simulink model "pedal_project"  (R2025b)
settings: Solver=VariableStepAuto  StartTime=0.0  StopTime=10.0  RelTol=1e-3
(part 2 of 2)

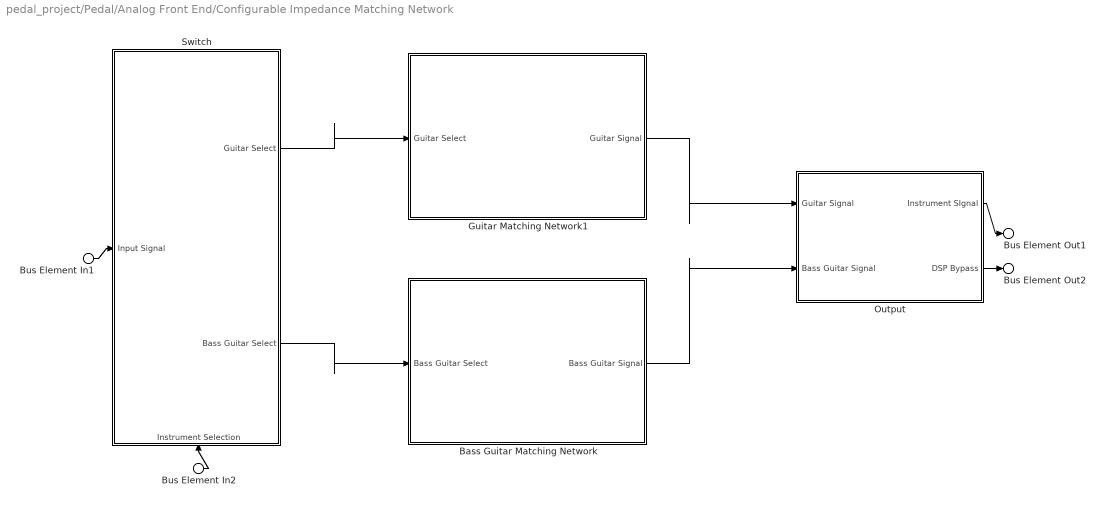
== system pedal_project/Pedal/Analog Front End/Configurable Impedance Matching Network ==
  Bus Element In2 : Inport  PortName=Instrument Selection
  Bus Element In1 : Inport  Port=2  PortName=Input Signal
  Bass Guitar Matching Network : Subsystem
      settings: PortSchema="{\"entries\":[{\"content\":{\"headerSize\":26,\"margin\":15,\"minimumSpacing\":25,\"sides\":[{\"content\":{\"connectorIds\":[\"In1\"]},\"type\":\"ConnectorPlacement.EquallySpacedRectSide\",\"uuid\":\"d45e420a-c48a-4f64-96ce-c5c35bb4ca1a\"},{\"content\":{\"connectorIds\":[\"Out1\"],\"side\":\"RIGHT\"},\"type\":\"ConnectorPlacement.EquallySpacedRectSide\",\"uuid\":\"a4e2bce0-d957-4e8d-907b-26e945724fec\"},{\"content\":{\"side\":\"TOP\"},\"type\":\"ConnectorPlacement.EquallySpacedRectSide\",\"uuid\":\"f887741f-84ea-4dc9-b916-61633ba77119\"}]},\"type\":\"ConnectorPlacement.EquallySpacedConnector\",\"uuid\":\"ffda6ec7-3a8c-4734-85c7-d4d2baf408ab\"}],\"packageUris\":[\"http://schema.mathworks.com/mf0/Connector/R2020b\"],\"version\":\"1.0\"}"
  Guitar Matching Network1 : Subsystem
      settings: PortSchema="{\"entries\":[{\"content\":{\"headerSize\":26,\"margin\":15,\"minimumSpacing\":25,\"sides\":[{\"content\":{\"connectorIds\":[\"In1\"]},\"type\":\"ConnectorPlacement.EquallySpacedRectSide\",\"uuid\":\"d45e420a-c48a-4f64-96ce-c5c35bb4ca1a\"},{\"content\":{\"connectorIds\":[\"Out1\"],\"side\":\"RIGHT\"},\"type\":\"ConnectorPlacement.EquallySpacedRectSide\",\"uuid\":\"a4e2bce0-d957-4e8d-907b-26e945724fec\"},{\"content\":{\"side\":\"TOP\"},\"type\":\"ConnectorPlacement.EquallySpacedRectSide\",\"uuid\":\"f887741f-84ea-4dc9-b916-61633ba77119\"}]},\"type\":\"ConnectorPlacement.EquallySpacedConnector\",\"uuid\":\"ffda6ec7-3a8c-4734-85c7-d4d2baf408ab\"}],\"packageUris\":[\"http://schema.mathworks.com/mf0/Connector/R2020b\"],\"version\":\"1.0\"}"
  Output : Subsystem
      settings: PortSchema="{\"entries\":[{\"content\":{\"headerSize\":26,\"margin\":15,\"minimumSpacing\":25,\"sides\":[{\"content\":{\"connectorIds\":[\"In1\",\"In2\"]},\"type\":\"ConnectorPlacement.EquallySpacedRectSide\",\"uuid\":\"d45e420a-c48a-4f64-96ce-c5c35bb4ca1a\"},{\"content\":{\"connectorIds\":[\"Out1\",\"Out2\"],\"side\":\"RIGHT\"},\"type\":\"ConnectorPlacement.EquallySpacedRectSide\",\"uuid\":\"a4e2bce0-d957-4e8d-907b-26e945724fec\"},{\"content\":{\"side\":\"TOP\"},\"type\":\"ConnectorPlacement.EquallySpacedRectSide\",\"uuid\":\"f887741f-84ea-4dc9-b916-61633ba77119\"}]},\"type\":\"ConnectorPlacement.EquallySpacedConnector\",\"uuid\":\"ffda6ec7-3a8c-4734-85c7-d4d2baf408ab\"}],\"packageUris\":[\"http://schema.mathworks.com/mf0/Connector/R2020b\"],\"version\":\"1.0\"}"
  Switch : Subsystem
      settings: PortSchema="{\"entries\":[{\"content\":{\"headerSize\":26,\"margin\":15,\"minimumSpacing\":25,\"sides\":[{\"content\":{\"connectorIds\":[\"In2\"]},\"type\":\"ConnectorPlacement.EquallySpacedRectSide\",\"uuid\":\"d45e420a-c48a-4f64-96ce-c5c35bb4ca1a\"},{\"content\":{\"connectorIds\":[\"Out1\",\"Out2\"],\"side\":\"RIGHT\"},\"type\":\"ConnectorPlacement.EquallySpacedRectSide\",\"uuid\":\"a4e2bce0-d957-4e8d-907b-26e945724fec\"},{\"content\":{\"side\":\"TOP\"},\"type\":\"ConnectorPlacement.EquallySpacedRectSide\",\"uuid\":\"f887741f-84ea-4dc9-b916-61633ba77119\"},{\"content\":{\"connectorIds\":[\"In1\"],\"side\":\"BOTTOM\"},\"type\":\"ConnectorPlacement.EquallySpacedRectSide\",\"uuid\":\"dfd7a217-587e-4736-a22e-6266921a1acc\"}]},\"type\":\"ConnectorPlacement.EquallySpacedConnector\",\"uuid\":\"ffda6ec7-3a8c-4734-85c7-d4d2baf408ab\"}],\"packageUris\":[\"http://schema.mathworks.com/mf0/Connector/R2020b\"],\"version\":\"1.0\"}"
  Bus Element Out1 : Outport  PortName=Instrument SIgnal
  Bus Element Out2 : Outport  Port=2  PortName=DSP Bypass
  wires:
  Bus Element In1/1 -> Switch/2(Input Signal)
  Switch/1(Guitar Select) -> Guitar Matching Network1/1(Guitar Select)
  Switch/2(Bass Guitar Select) -> Bass Guitar Matching Network/1(Bass Guitar Select)
  Bus Element In2/1 -> Switch/1(Instrument Selection)
  Output/1(Instrument SIgnal) -> Bus Element Out1/1
  Guitar Matching Network1/1(Guitar Signal) -> Output/1(Guitar Signal)
  Bass Guitar Matching Network/1(Bass Guitar Signal) -> Output/2(Bass Guitar Signal)
  Output/2(DSP Bypass) -> Bus Element Out2/1

== system pedal_project/Pedal/Analog Signal Processing/1//4 Inch TS Input Jack1 ==
  Bus Element In1 : Inport  PortName=Post Extern Sig
  Bus Element Out1 : Outport  PortName=External Signal

== system pedal_project/Pedal/Analog Signal Processing/1//4 Inch TS Ouput Jack ==
  Bus Element In1 : Inport  PortName=Extern Sig Input
  Bus Element Out1 : Outport  PortName=Post DSP Sig

== system pedal_project/Pedal/Analog Signal Processing/Analog Processing Network ==
  Bus Element In3 : Inport  PortName=Post Extern Sig
  Bus Element In1 : Inport  Port=2  PortName=ASP Effects Power
  Bus Element In2 : Inport  Port=3  PortName=Analog Chain Config
  Bus Element Out1 : Outport  PortName=Post ASP Sig

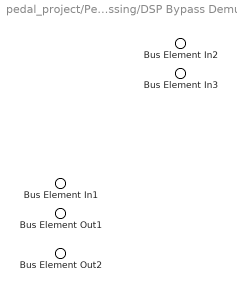
== system pedal_project/Pedal/Analog Signal Processing/DSP Bypass Demux ==
  Bus Element In3 : Inport  PortName=DSP Bypass Config
  Bus Element In2 : Inport  Port=2  PortName=DSP Bypass
  Bus Element In1 : Inport  Port=3  PortName=DSP Signal
  Bus Element Out1 : Outport  PortName=Extern Sig Input
  Bus Element Out2 : Outport  Port=2  PortName=Extern Bypass Sig

== system pedal_project/Pedal/Analog Signal Processing/Extern Bypass Demux ==
  Bus Element In2 : Inport  PortName=Extern Bypass Sig
  Bus Element In1 : Inport  Port=2  PortName=External Signal
  Bus Element Out1 : Outport  PortName=Post Extern Sig

== system pedal_project/Pedal/Control/Dial//Switch Network ==
  Bus Element Out1 : Outport  PortName=Parameters Config

== system pedal_project/Pedal/Control/Input Type Selector ==
  Bus Element Out1 : Outport  PortName=Instrument Selection

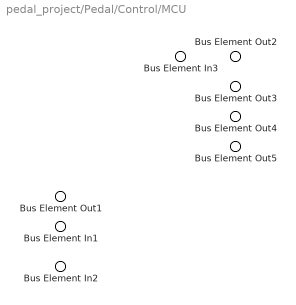
== system pedal_project/Pedal/Control/MCU ==
  Bus Element In3 : Inport  PortName=MCU Power
  Bus Element In1 : Inport  Port=2  PortName=Parameters Config
  Bus Element In2 : Inport  Port=3  PortName=Configuration Packets
  Bus Element Out5 : Outport  PortName=ASP Bypass Config
  Bus Element Out4 : Outport  Port=2  PortName=Preamp Bypass
  Bus Element Out3 : Outport  Port=3  PortName=DSP Bypass Config
  Bus Element Out2 : Outport  Port=4  PortName=Analog Chain Config
  Bus Element Out1 : Outport  Port=5  PortName=DSP Config

== system pedal_project/Pedal/Control/USB Port ==
  Bus Element In1 : Inport  PortName=App Control Packets
  Bus Element Out1 : Outport  PortName=Configuration Packets

== system pedal_project/Pedal/Digital Signal Processing/40 kHz LPF ==
  Bus Element In1 : Inport  PortName=DSP Output Sig
  Bus Element Out1 : Outport  PortName=DSP Signal
  Bus Element Out2 : Outport  Port=2  PortName=ASP Bypass

== system pedal_project/Pedal/Digital Signal Processing/DSP Core ==
  Bus Element In3 : Inport  PortName=DSP Config
  Bus Element In2 : Inport  Port=2  PortName=DSP Core Power
  Bus Element In1 : Inport  Port=3  PortName=Instrument SIgnal
  Bus Element Out1 : Outport  PortName=DSP Output Sig

== system pedal_project/Pedal/Electronics Power Distribution/9V 2.1mm Jack ==
  Bus Element In1 : Inport  PortName=9V DC
  Bus Element Out1 : Outport  PortName=DC In

== system pedal_project/Pedal/Electronics Power Distribution/Power Bus ==
  Bus Element In1 : Inport  PortName=DC In
  Bus Element Out2 : Outport  PortName=DSP Core Power
  Bus Element Out3 : Outport  Port=2  PortName=ASP Effects Power
  Bus Element Out1 : Outport  Port=3  PortName=MCU Power

== system pedal_project/Pedal/Output Drivers/1//4 Inch TS Ouput ==
  Bus Element In1 : Inport  PortName=Amp Sig
  Bus Element Out1 : Outport  PortName=TS Out

== system pedal_project/Pedal/Output Drivers/1//8 Inch TRS Ouput ==
  Bus Element In1 : Inport  PortName=Amp TRS Sig
  Bus Element Out1 : Outport  PortName=TRS Out

== system pedal_project/Pedal/Output Drivers/ASP Bypass Demux ==
  Bus Element In3 : Inport  PortName=ASP Bypass Config
  Bus Element In2 : Inport  Port=2  PortName=Post ASP Sig
  Bus Element In1 : Inport  Port=3  PortName=ASP Bypass
  Bus Element Out1 : Outport  PortName=ASP Sig

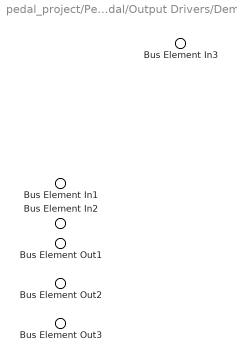
== system pedal_project/Pedal/Output Drivers/Demux ==
  Bus Element In1 : Inport  PortName=Amplified Signal
  Bus Element In3 : Inport  Port=2  PortName=Bypass Sig
  Bus Element In2 : Inport  Port=3  PortName=Preamp Bypass
  Bus Element Out1 : Outport  PortName=Amp TS Sig
  Bus Element Out2 : Outport  Port=2  PortName=Amp XLR Sig
  Bus Element Out3 : Outport  Port=3  PortName=Amp TRS Sig

== system pedal_project/Pedal/Output Drivers/Out Bus ==
  Bus Element In4 : Inport  PortName=MIDI Sig
  Bus Element In1 : Inport  Port=2  PortName=TS Out
  Bus Element In2 : Inport  Port=3  PortName=XLR Out
  Bus Element In3 : Inport  Port=4  PortName=TRS Out
  Bus Element Out1 : Outport  PortName=Audio Signal Output

== system pedal_project/Pedal/Output Drivers/Preamp ==
  Bus Element In1 : Inport  PortName=Preamp Sig
  Bus Element Out1 : Outport  PortName=Amplified Signal

== system pedal_project/Pedal/Output Drivers/Sig Combiner ==
  Bus Element In1 : Inport  PortName=ASP Sig
  Bus Element Out3 : Outport  PortName=Bypass Sig
  Bus Element Out2 : Outport  Port=2  PortName=Preamp Sig
  Bus Element Out1 : Outport  Port=3  PortName=USB MIDI Sig

== system pedal_project/Pedal/Output Drivers/USB MIDI ==
  Bus Element In1 : Inport  PortName=USB MIDI Sig
  Bus Element Out1 : Outport  PortName=MIDI Sig

== system pedal_project/Pedal/Output Drivers/XLR Ouput ==
  Bus Element In1 : Inport  PortName=Amp XLR Sig
  Bus Element Out1 : Outport  PortName=XLR Out

== system pedal_project/Phone/Software Application/Configurable Analog Processing ==
  Bus Element Out1 : Outport  PortName=Analog Effects Configuration

== system pedal_project/Phone/Software Application/Configurable Digital Processing ==
  Bus Element Out1 : Outport  PortName=Digital Effects Configuration

== system pedal_project/Phone/Software Application/Effects Validation and Upload ==
  Bus Element In1 : Inport  PortName=Analog Effects Configuration
  Bus Element In2 : Inport  Port=2  PortName=Digital Effects Configuration
  Bus Element Out1 : Outport  PortName=Configuration Upload Packets

== system pedal_project/Pedal/Analog Front End/Configurable Impedance Matching Network/Bass Guitar Matching Network ==
  Bus Element In1 : Inport  PortName=Bass Guitar Select
  Bus Element Out1 : Outport  PortName=Bass Guitar Signal

== system pedal_project/Pedal/Analog Front End/Configurable Impedance Matching Network/Guitar Matching Network1 ==
  Bus Element In1 : Inport  PortName=Guitar Select
  Bus Element Out1 : Outport  PortName=Guitar Signal

== system pedal_project/Pedal/Analog Front End/Configurable Impedance Matching Network/Output ==
  Bus Element In1 : Inport  PortName=Guitar Signal
  Bus Element In2 : Inport  Port=2  PortName=Bass Guitar Signal
  Bus Element Out1 : Outport  PortName=Instrument SIgnal
  Bus Element Out2 : Outport  Port=2  PortName=DSP Bypass

== system pedal_project/Pedal/Analog Front End/Configurable Impedance Matching Network/Switch ==
  Bus Element In2 : Inport  PortName=Instrument Selection
  Bus Element In1 : Inport  Port=2  PortName=Input Signal
  Bus Element Out1 : Outport  PortName=Guitar Select
  Bus Element Out2 : Outport  Port=2  PortName=Bass Guitar Select
